simulink model "AC_AFCS"  (R2021b)
settings: Solver=VariableStepAuto  StartTime=0.0  StopTime=1000  RelTol=1e-3
values from neighbouring files (symbols this model uses):
  ss_red = ss(A_ac1, B_ac1, C_ac1, D_ac1, 'StateName', SS_long_lo.StateName(states_lon2),      'InputName', SS_long_lo.InputName(inputs_lon2), 'OutputName', SS_long_lo.OutputName(outputs_lon2))    [chap8.m]
  trim_control_lo = [-2.46068617229 4.27328139671e-15 3.64793526166e-14]    [15000_500_lin.mat]    (also in 20000_600_lin.mat = [-2.20565803063 -5.72373630956e-15 -2.7298127136e-14]; 20000_700_lin.mat = [-1.89781127963 4.04049856894e-15 1.70583711485e-14]; 20000_900_lin.mat = [-1.56151521394 5.64609304487e-14 2.61420891923e-13]; chapter8.mat = [-4.18911302139 -1.99262868586e-15 1.24058797748e-14])
  trim_state_lo = [0 0 15000 0 0.0779375118365 0 500 0.0779375118365 0 0 0 0]    [15000_500_lin.mat]    (also in 20000_600_lin.mat = [0 0 20000 0 0.0594178286879 0 600 0.0594178286879 0 0 0 0]; 20000_700_lin.mat = [0 0 20000 0 0.0369748641994 0 700 0.0369748641994 0 0 0 0]; 20000_900_lin.mat = [0 0 20000 0 0.0123475459982 0 900 0.0123475459982 0 0 0 0]; chapter8.mat = [0 0 5000 0 0.182405640343 0 300 0.182405640343 0 0 0 0])
  trim_thrust_lo = 2120.62144782    [15000_500_lin.mat]    (also in 20000_600_lin.mat = 2085.07224914; 20000_700_lin.mat = 2312.58724711; 20000_900_lin.mat = 3496.52746761; chapter8.mat = 2826.8165433)
libraries: simulink_extras x3, slpidlib x3
settings Model: Creator=wardb  LastModifiedBy=wardb
settings SolverCC: AlgebraicLoopSolver=TrustRegion
settings DebuggingCC: SFMachineParentedDataDiag=warning

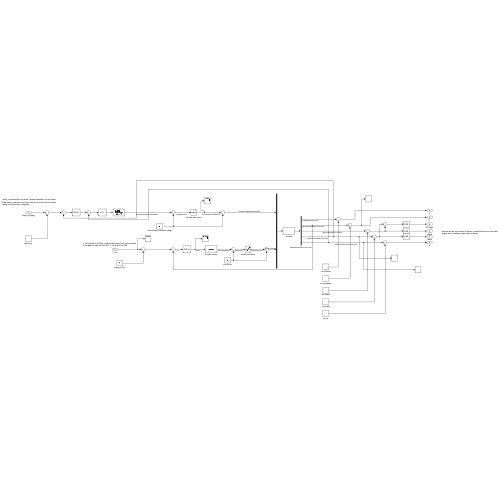
[thumbnail: Simulink's stored preview of the top-level diagram]
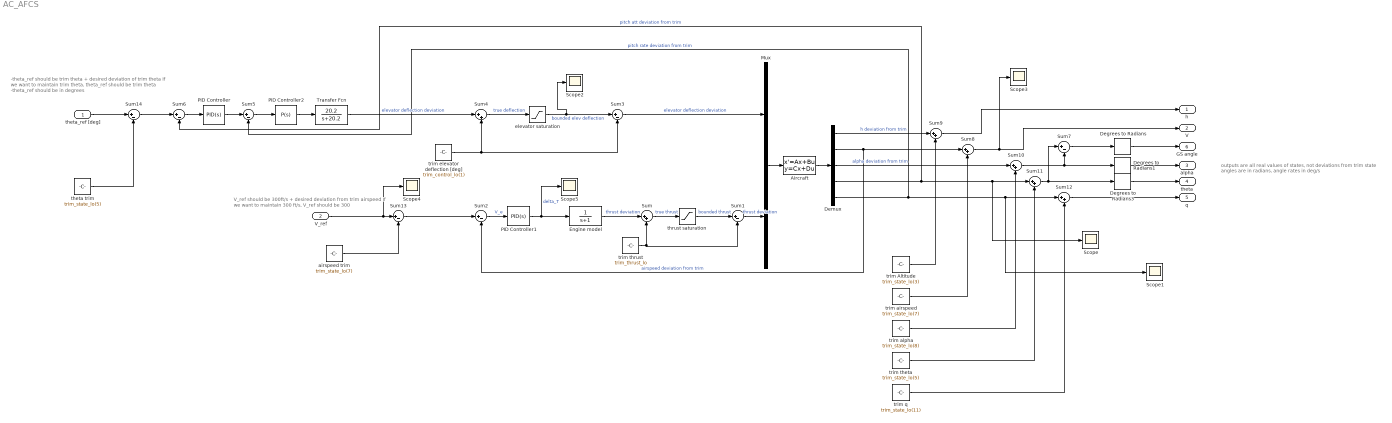
== system AC_AFCS ==
  note: -theta_ref should be trim theta + desired deviation of trim theta
      | If we want to maintain trim theta, theta_ref should be trim theta
      | -theta_ref should be in degrees
  note: outputs are all real values of states, not deviations from trim state
      | angles are in radians, angle rates in deg/s
  note: V_ref should be 300ft/s + desired deviation from trim airspeed
      | If we want to maintain 300 ft/s, V_ref should be 300
  theta_ref [deg] : Inport
  V_ref : Inport  Port=2
  Aircraft : StateSpace  A=ss_red.A  B=ss_red.B  C=ss_red.C  D=ss_red.D  InitialCondition=0
  Degrees to Radians : simulink_extras/Transformations/Degrees to Radians
  Degrees to Radians1 : simulink_extras/Transformations/Degrees to Radians
  Degrees to Radians3 : simulink_extras/Transformations/Degrees to Radians
  Demux : Demux  Outputs=5
  Engine model : TransferFcn  Denominator=[1 1]
  Mux : Mux  Inputs=2
  PID Controller : slpidlib/PID Controller  Controller=PID  Form=Parallel  TimeDomain=Continuous-time  UseExternalTs=off  SampleTime=-1  IntegratorMethod=Forward Euler  FilterMethod=Forward Euler  ControllerParametersSource=internal  P=0.126869189059665  I=5.34397207151188e-07  D=3191.97869211359  UseFilter=on  N=0.0068326230933842  TunerSelectOption=Transfer Function Based (PID Tuner App)  InitialConditionSource=internal  InitialConditionForIntegrator=0  InitialConditionForFilter=0  DifferentiatorICPrevScaledInput=0  ExternalReset=none  TrackingMode=off  Kt=1  LimitOutput=off  SatLimitsSource=internal  UpperSaturationLimit=inf  LowerSaturationLimit=-inf  LinearizeAsGain=on  AntiWindupMode=none  Kb=1  POutMin=[]  POutMax=[]  IOutMin=[]  IOutMax=[]  DOutMin=[]  DOutMax=[]  NOutMin=[]  NOutMax=[]  SumOutMin=[]  SumOutMax=[]  SaturationOutMin=[]  SaturationOutMax=[]  PParamMin=[]  PParamMax=[]  IParamMin=[]  IParamMax=[]  DParamMin=[]  DParamMax=[]  NParamMin=[]  NParamMax=[]  KbParamMin=[]  KbParamMax=[]  KtParamMin=[]  KtParamMax=[]  KbOutMin=[]  KbOutMax=[]  KtOutMin=[]  KtOutMax=[]  IntegratorOutMin=[]  IntegratorOutMax=[]  FilterOutMin=[]  FilterOutMax=[]  SumI1OutMin=[]  SumI1OutMax=[]  SumI2OutMin=[]  SumI2OutMax=[]  SumI3OutMin=[]  SumI3OutMax=[]  SumI4OutMin=[]  SumI4OutMax=[]  SumDOutMin=[]  SumDOutMax=[]  DifferentiatorOutMin=[]  DifferentiatorOutMax=[]  FilterDiffOutCoefMin=[]  FilterDiffOutCoefMax=[]  ReciprocalOutMin=[]  ReciprocalOutMax=[]  SumDenOutMin=[]  SumDenOutMax=[]  SumNumOutMin=[]  SumNumOutMax=[]  DivideOutMin=[]  DivideOutMax=[]  UdiffTsProdOutMin=[]  UdiffTsProdOutMax=[]  NTsProdOutMin=[]  NTsProdOutMax=[]  UintegralTsProdOutMin=[]  UintegralTsProdOutMax=[]  UngainTsProdOutMin=[]  UngainTsProdOutMax=[]  IntegratorContinuousStateAttributes=''  IntegratorStateMustResolveToSignalObject=off  IntegratorRTWStateStorageClass=Auto  FilterContinuousStateAttributes=''  FilterStateMustResolveToSignalObject=off  FilterRTWStateStorageClass=Auto  ParallelPVariant=InternalParameters  IdealPVariant=Disabled  IVariant=InternalParameters  DVariant=InternalParameters  IntegratorVariant=Continuous  SatVariant=Disabled  AWVariant=Passthrough  PCopyVariant=Disabled  TRVariant=Disabled  FdbkBlocksVariant=Forward  IdealPFdbkVariant=Disabled  SatFdbkVariant=Disabled  DerivativeFilterVariant=ContFilter  NVariant=InternalParameters  NCopyVariant=Disabled  FilterICVariant=InternalICsFilter  IntegratorICVariant=InternalICs  ExternalResetVariant=Disabled  TRSumVariant=Passthrough  SumFdbkVariant=Disabled  SumVariant=Sum_PID  TsampFilterVariant=InternalTs  TsampNgainVariant=Passthrough  TsampIntegralVariant=Passthrough  ExternalSaturationOutDataTypeStr=Inherit: Same as second input
  PID Controller1 : slpidlib/PID Controller  Controller=PID  Form=Parallel  TimeDomain=Continuous-time  UseExternalTs=off  SampleTime=-1  IntegratorMethod=Forward Euler  FilterMethod=Forward Euler  ControllerParametersSource=internal  P=100.544379315609  I=6.08761343845027  D=-35.7772852997847  UseFilter=on  N=0.158620786783013  TunerSelectOption=Transfer Function Based (PID Tuner App)  InitialConditionSource=internal  InitialConditionForIntegrator=0  InitialConditionForFilter=0  DifferentiatorICPrevScaledInput=0  ExternalReset=none  TrackingMode=off  Kt=1  LimitOutput=off  SatLimitsSource=internal  UpperSaturationLimit=inf  LowerSaturationLimit=-inf  LinearizeAsGain=on  AntiWindupMode=none  Kb=1  POutMin=[]  POutMax=[]  IOutMin=[]  IOutMax=[]  DOutMin=[]  DOutMax=[]  NOutMin=[]  NOutMax=[]  SumOutMin=[]  SumOutMax=[]  SaturationOutMin=[]  SaturationOutMax=[]  PParamMin=[]  PParamMax=[]  IParamMin=[]  IParamMax=[]  DParamMin=[]  DParamMax=[]  NParamMin=[]  NParamMax=[]  KbParamMin=[]  KbParamMax=[]  KtParamMin=[]  KtParamMax=[]  KbOutMin=[]  KbOutMax=[]  KtOutMin=[]  KtOutMax=[]  IntegratorOutMin=[]  IntegratorOutMax=[]  FilterOutMin=[]  FilterOutMax=[]  SumI1OutMin=[]  SumI1OutMax=[]  SumI2OutMin=[]  SumI2OutMax=[]  SumI3OutMin=[]  SumI3OutMax=[]  SumI4OutMin=[]  SumI4OutMax=[]  SumDOutMin=[]  SumDOutMax=[]  DifferentiatorOutMin=[]  DifferentiatorOutMax=[]  FilterDiffOutCoefMin=[]  FilterDiffOutCoefMax=[]  ReciprocalOutMin=[]  ReciprocalOutMax=[]  SumDenOutMin=[]  SumDenOutMax=[]  SumNumOutMin=[]  SumNumOutMax=[]  DivideOutMin=[]  DivideOutMax=[]  UdiffTsProdOutMin=[]  UdiffTsProdOutMax=[]  NTsProdOutMin=[]  NTsProdOutMax=[]  UintegralTsProdOutMin=[]  UintegralTsProdOutMax=[]  UngainTsProdOutMin=[]  UngainTsProdOutMax=[]  IntegratorContinuousStateAttributes=''  IntegratorStateMustResolveToSignalObject=off  IntegratorRTWStateStorageClass=Auto  FilterContinuousStateAttributes=''  FilterStateMustResolveToSignalObject=off  FilterRTWStateStorageClass=Auto  ParallelPVariant=InternalParameters  IdealPVariant=Disabled  IVariant=InternalParameters  DVariant=InternalParameters  IntegratorVariant=Continuous  SatVariant=Disabled  AWVariant=Passthrough  PCopyVariant=Disabled  TRVariant=Disabled  FdbkBlocksVariant=Forward  IdealPFdbkVariant=Disabled  SatFdbkVariant=Disabled  DerivativeFilterVariant=ContFilter  NVariant=InternalParameters  NCopyVariant=Disabled  FilterICVariant=InternalICsFilter  IntegratorICVariant=InternalICs  ExternalResetVariant=Disabled  TRSumVariant=Passthrough  SumFdbkVariant=Disabled  SumVariant=Sum_PID  TsampFilterVariant=InternalTs  TsampNgainVariant=Passthrough  TsampIntegralVariant=Passthrough  ExternalSaturationOutDataTypeStr=Inherit: Same as second input
  PID Controller2 : slpidlib/PID Controller  Controller=P  Form=Parallel  TimeDomain=Continuous-time  UseExternalTs=off  SampleTime=-1  IntegratorMethod=Forward Euler  FilterMethod=Forward Euler  ControllerParametersSource=internal  P=-0.0635335950698202  I=1  D=0  UseFilter=on  N=100  TunerSelectOption=Transfer Function Based (PID Tuner App)  InitialConditionSource=internal  InitialConditionForIntegrator=0  InitialConditionForFilter=0  DifferentiatorICPrevScaledInput=0  ExternalReset=none  TrackingMode=off  Kt=1  LimitOutput=off  SatLimitsSource=internal  UpperSaturationLimit=inf  LowerSaturationLimit=-inf  LinearizeAsGain=on  AntiWindupMode=none  Kb=1  POutMin=[]  POutMax=[]  IOutMin=[]  IOutMax=[]  DOutMin=[]  DOutMax=[]  NOutMin=[]  NOutMax=[]  SumOutMin=[]  SumOutMax=[]  SaturationOutMin=[]  SaturationOutMax=[]  PParamMin=[]  PParamMax=[]  IParamMin=[]  IParamMax=[]  DParamMin=[]  DParamMax=[]  NParamMin=[]  NParamMax=[]  KbParamMin=[]  KbParamMax=[]  KtParamMin=[]  KtParamMax=[]  KbOutMin=[]  KbOutMax=[]  KtOutMin=[]  KtOutMax=[]  IntegratorOutMin=[]  IntegratorOutMax=[]  FilterOutMin=[]  FilterOutMax=[]  SumI1OutMin=[]  SumI1OutMax=[]  SumI2OutMin=[]  SumI2OutMax=[]  SumI3OutMin=[]  SumI3OutMax=[]  SumI4OutMin=[]  SumI4OutMax=[]  SumDOutMin=[]  SumDOutMax=[]  DifferentiatorOutMin=[]  DifferentiatorOutMax=[]  FilterDiffOutCoefMin=[]  FilterDiffOutCoefMax=[]  ReciprocalOutMin=[]  ReciprocalOutMax=[]  SumDenOutMin=[]  SumDenOutMax=[]  SumNumOutMin=[]  SumNumOutMax=[]  DivideOutMin=[]  DivideOutMax=[]  UdiffTsProdOutMin=[]  UdiffTsProdOutMax=[]  NTsProdOutMin=[]  NTsProdOutMax=[]  UintegralTsProdOutMin=[]  UintegralTsProdOutMax=[]  UngainTsProdOutMin=[]  UngainTsProdOutMax=[]  IntegratorContinuousStateAttributes=''  IntegratorStateMustResolveToSignalObject=off  IntegratorRTWStateStorageClass=Auto  FilterContinuousStateAttributes=''  FilterStateMustResolveToSignalObject=off  FilterRTWStateStorageClass=Auto  ParallelPVariant=InternalParameters  IdealPVariant=Disabled  IVariant=Disabled  DVariant=Disabled  IntegratorVariant=Disabled  SatVariant=Disabled  AWVariant=Disabled  PCopyVariant=Disabled  TRVariant=Disabled  FdbkBlocksVariant=Forward  IdealPFdbkVariant=Disabled  SatFdbkVariant=Disabled  DerivativeFilterVariant=Disabled  NVariant=Disabled  NCopyVariant=Disabled_SignalSpec  FilterICVariant=Disabled  IntegratorICVariant=Disabled  ExternalResetVariant=Disabled  TRSumVariant=Passthrough  SumFdbkVariant=Disabled  SumVariant=Passthrough_P  TsampFilterVariant=InternalTs  TsampNgainVariant=Passthrough  TsampIntegralVariant=Disabled_SignalSpec  ExternalSaturationOutDataTypeStr=Inherit: Same as second input
  Scope{,1..5} (6 alike) : Scope
  Sum{,4,8..12} (7 alike) : Sum  Inputs=|++
  Sum{1..3,5..7,13..14} (8 alike) : Sum  Inputs=|+-
  Transfer Fcn : TransferFcn  Numerator=[20.2]  Denominator=[1, 20.2]
  airspeed trim : Constant  Value=trim_state_lo(7)
  elevator saturation : Saturate  UpperLimit=25  LowerLimit=-25
  theta trim : Constant  Value=trim_state_lo(5)
  thrust saturation : Saturate  UpperLimit=19000  LowerLimit=1000
  trim Altitude : Constant  Value=trim_state_lo(3)
  trim airspeed : Constant  Value=trim_state_lo(7)
  trim alpha : Constant  Value=trim_state_lo(8)
  trim elevator deflection [deg] : Constant  Value=trim_control_lo(1)
  trim q : Constant  Value=trim_state_lo(11)
  trim theta : Constant  Value=trim_state_lo(5)
  trim thrust : Constant  Value=trim_thrust_lo
  h : Outport
  V : Outport  Port=2
  alpha : Outport  Port=3
  theta : Outport  Port=4
  q : Outport  Port=5
  GS angle : Outport  Port=6
  wires:
  trim alpha/1 -> Sum10/2
  trim thrust/1 -> Sum1/2, Sum/2
  trim Altitude/1 -> Sum9/2
  Degrees to Radians3/1 -> theta/1
  Demux/1 -> Sum9/1  "h deviation from trim"
  Sum13/1 -> Sum2/1
  theta trim/1 -> Sum14/2
  PID Controller/1 -> Sum5/1
  PID Controller2/1 -> Transfer Fcn/1
  airspeed trim/1 -> Sum13/2
  Sum4/1 -> elevator saturation/1  "true deflection"
  Demux/4 -> Sum6/2, Scope/1, Sum11/1  "pitch att deviation from trim"
  Sum14/1 -> Sum6/1
  Degrees to Radians1/1 -> alpha/1
  Sum6/1 -> PID Controller/1
  Sum5/1 -> PID Controller2/1
  Engine model/1 -> Sum/1  "thrust deviation"
  trim q/1 -> Sum12/2
  Transfer Fcn/1 -> Sum4/1  "elevator deflection deviation"
  Sum10/1 -> Degrees to Radians1/1, Sum7/2
  Sum7/1 -> Degrees to Radians/1
  Sum12/1 -> q/1
  Sum11/1 -> Degrees to Radians3/1, Sum7/1
  Sum8/1 -> Scope3/1, V/1
  trim elevator deflection [deg]/1 -> Sum3/2, Sum4/2
  elevator saturation/1 -> Scope2/1, Sum3/1  "bounded elev deflection"
  Demux/3 -> Sum10/1  "alpha deviation from trim"
  Degrees to Radians/1 -> GS angle/1
  Sum2/1 -> PID Controller1/1  "V_e"
  trim airspeed/1 -> Sum8/2
  Demux/5 -> Sum5/2, Scope1/1, Sum12/1  "pitch rate deviation from trim"
  Aircraft/1 -> Demux/1
  theta_ref [deg]/1 -> Sum14/1
  PID Controller1/1 -> Scope5/1, Engine model/1  "delta_T"
  Sum1/1 -> Mux/2  "thrust deviation"
  Sum9/1 -> h/1
  thrust saturation/1 -> Sum1/1  "bounded thrust"
  Sum3/1 -> Mux/1  "elevator deflection deviation"
  Mux/1 -> Aircraft/1
  Sum/1 -> thrust saturation/1  "true thrust"
  Demux/2 -> Sum8/1, Sum2/2  "airspeed deviation from trim"
  trim theta/1 -> Sum11/2
  V_ref/1 -> Sum13/1, Scope4/1
